simulink model "controlMCUCalibrateSurfaces"  (Simulink 6.6)
settings: Solver=FixedStepDiscrete  StartTime=0.0  StopTime=10.0  FixedStep=0.01  RelTol=1e-3
InitFcn:
  | mcuInit
undefined symbols (not defined in the file or in its folder): bdr, controlMCUInit, getPidIdx, gsRead, mdr, pilotCommands, prepareTelemetry, protParseDecode, protParseDecodeGS, readIpc, send2GS, u1, updateLoad, updatePWM, y1
libraries: dsPICdrivers x21, aerolibconvert2 x1, simulink x1
settings Model: Creator=ASL_Lab  LastModifiedBy=Administrator  ProdHWDeviceType=16-bit Generic
settings OptimizationCC: InlineParams=on  OptimizeModelRefInitCode=on  LifeSpan=1
settings HardwareCC: ProdBitPerInt=16  ProdEndianess=LittleEndian  ProdWordSize=16  ProdHWDeviceType=16-bit Generic  TargetHWDeviceType=32-bit Generic
settings RTWCC: SystemTargetFile=dspic.tlc  TemplateMakefile=dspic_pic30_gcc.tmf  PostCodeGenCommand=dsPIC_Compile()  Description=Embedded Target for Microchip dsPIC (real-time)  GenerateReport=on  ProcessScript=dspic_make_rtw_hook  IncludeHyperlinkInReport=on  LaunchReport=on
settings RTWCC: CustomSource=|
  | clib\circBuffer.c
  | clib\gpsSplit.c
  | clib\sbrk.c
  | clib\interProcCommSlave.c
  | clib\sendProtocol.c
  | clib\protDecoder.c
  | clib\groundStationDriver.c
  | clib\apUtils.c
  | clib\DEE.c
  | clib\DEES.s
  | clib\navSupport.c
settings CodeAppCC: IgnoreCustomStorageClasses=off
settings STFCustomTargetCC: TargetFcnLib=ansi_tfl_tmw.mat  GenFloatMathFcnCalls=ANSI_C  ModelReferenceCompliant=off  IncludeMdlTerminateFcn=off  CombineOutputUpdateFcns=on  SuppressErrorStatus=on  ERTCustomFileBanners=on  SupportContinuousTime=off  SupportNonInlinedSFcns=off  SystemTargetFile=dspic.tlc
settings ERTTargetCC: TargetFcnLib=ansi_tfl_tmw.mat  GenFloatMathFcnCalls=ANSI_C  ModelReferenceCompliant=off  IncludeMdlTerminateFcn=off  SuppressErrorStatus=on  ModelStepFunctionPrototypeControlCompliant=off  ExtModeMexFile=noextcomm  InlinedParameterPlacement=NonHierarchical  ERTSrcFileBannerTemplate=dsPIC_code_template.cgt  ERTHdrFileBannerTemplate=dsPIC_code_template.cgt  ERTDataSrcFileTemplate=dsPIC_code_template.cgt  ERTDataHdrFileTemplate=dsPIC_code_template.cgt  ERTCustomFileTemplate=dsPIC_main.tlc
settings CustomProperty: DataType=string  Value=C:\PROGRA~1\MATLAB\R2007a\rtw\bin\win32\gmake

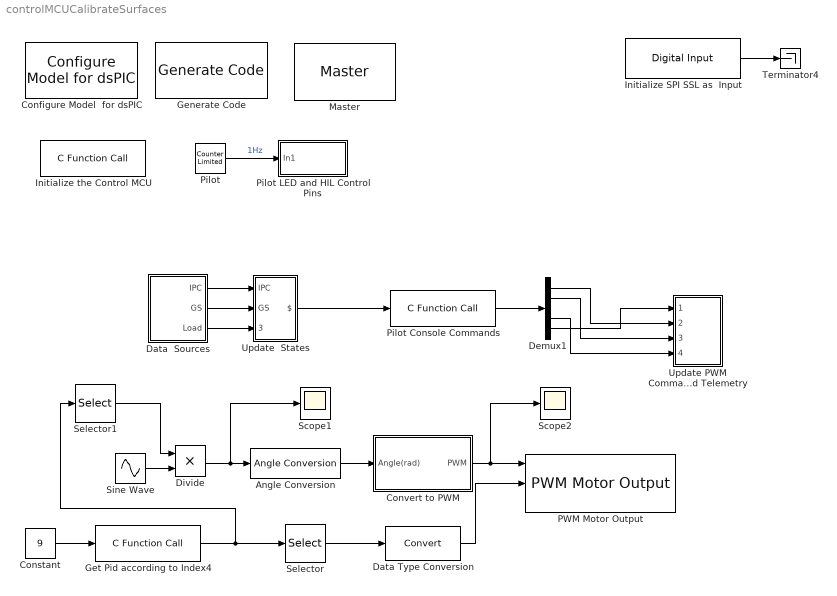
== system controlMCUCalibrateSurfaces ==
  Angle Conversion : aerolibconvert2/Angle Conversion  SystemSampleTime=-1  IU=deg  OU=rad
  Configure Model  for dsPIC : dsPICdrivers/Simulink Configuration/Configure Model  for dsPIC
  Constant : Constant  Value=9  OutDataTypeMode=uint8
  Convert to PWM : Subsystem  mask{slopem=mdr, interceptb=bdr}
      mask prompts: slopem "Slope"; interceptb "Intercept"
  Data  Sources : Subsystem
  Data Type Conversion : DataTypeConversion  OutDataTypeMode=uint16
  Demux1 : Demux  Outputs=5
  Divide : Product  OutScaling=2^-10
  Generate Code : dsPICdrivers/Simulink Configuration/Generate Code
  Get Pid according to Index4 : dsPICdrivers/OTHERS/C Function Call  Tag=dsPIC_dsPIC_CFunctionCall  fctName='getPidIdx'  INPUT_SIZE=1  INPUT1=uint8  INPUT2=--  INPUT3=--  OUTPUT_SIZE=3  OUTPUT1=real32  SampleTime=.01  InputType=[ 2 ]  OutputType=[ 7 ]  FctDeclaration=extern void getPidIdx(uint8_T u1,real32_T* y1);  FctCall=getPidIdx(%u1, *%y1);  OrderingInOutPopup=None
  Initialize SPI SSL as  Input : dsPICdrivers/Digital I//O/Digital Input  Tag=dsPIC_Digital_Input  PORT=B  Pin=[2]  SampleTime=inf  OrderingInOutPopup=None
  Initialize the Control MCU : dsPICdrivers/OTHERS/C Function Call  Tag=dsPIC_dsPIC_CFunctionCall  fctName='controlMCUInit'  INPUT_SIZE=1  INPUT1=--  INPUT2=--  INPUT3=--  OUTPUT_SIZE=1  OUTPUT1=--  SampleTime=inf  InputType=[ ]  OutputType=[ ]  FctDeclaration=extern void controlMCUInit();  FctCall=controlMCUInit();  OrderingInOutPopup=None
  Master : dsPICdrivers/Master  Tag=dsPIC_MASTER  Priority=1  TimeStepType=Timer1  picType=33fJ256MC710  fcy=40000000  Quartz_33f=12e6  PLLActive_33f=on  fcyDesired_33f=40e6  tmr1="[8  49999  0]"  tmr1Info="Time Step : 0.01  ;   Error : 0%  PR1=49999"  tmr2345="[0  0  0  0  0  0  0  0]"  tmr2345cfg=[-1 -1 -1 -1 -1 -1 -1 -1]  IOautoConf=on  typePort="[ 0   0   0   0   0   0   0   0   0   0   0   0   0   0   0   0   0   0   9   0   0   0  10  10   0   0   0   0   0   0   0   0   0   0   0   0   0   0   0   0   0   0   0   0   0   0   0   0   0   0   0   0   0   0   0   0   0   0   0   0   0   0   0   0  11   0   0   0  11   0  11   0   0  10   0   0   0   0   0   0   0   0   0   0   0   0   0   0   0   0   0   0   0   0   0   0   0   0   0   0   0   0   0   0   0   0   0   0   0   0   0   0 ]"  TRIS="[ 65535  65343  65535  65535  65023  65535  65535 ]"  ADPCFG=2097348  MasterBusyPort=None  MasterOverloadPort=None  FOSC=Quartz (XT - HS)  TempProtection_33f=TEMP_ON  FPBOR=<empty>  PWRT=64ms  MCLR=<empty>  PowerSave=off
  PWM Motor Output : dsPICdrivers/Peripheral I//O/PWM Motor Output  Tag=dsPIC_PWM_Motor  Priority=5  InputEnableChk=off  InputPeriodeChk=off  Channel=[1 3 4]  TPeriode=.02  PrescalerValue=16  PeriodeInteger=25000  MaxName='PWM'  Centered=on  HChannelON=off  Info="Nbr Bits : 15.6096  ||  PWM = 50000  ||  Prescaler = 16"  Delay=0  IntPriority=5  nbrPwmChannelPIC=4  Status=OK
  Pilot : simulink/Sources/Counter Limited  SystemSampleTime=-1  uplimit=1  tsamp=1.0
  Pilot Console Commands : dsPICdrivers/OTHERS/C Function Call  Tag=dsPIC_dsPIC_CFunctionCall  fctName='pilotCommands'  INPUT_SIZE=1  INPUT1=--  INPUT2=--  INPUT3=--  OUTPUT_SIZE=5  OUTPUT1=uint16  SampleTime=.01  InputType=[ ]  OutputType=[ 4 ]  FctDeclaration=extern void pilotCommands(uint16_T* y1);  FctCall=pilotCommands(*%y1);  OrderingInOutPopup=Input
  Pilot LED and HIL Control Pins : Subsystem
  Scope1 : Scope
  Scope2 : Scope
  Selector : Selector  IndexOptions=Index vector (dialog)  Indices=[1]  OutputSizes=1  InputPortWidth=3
  Selector1 : Selector  IndexOptions=Index vector (dialog)  Indices=[2]  OutputSizes=1  InputPortWidth=3
  Sine Wave : Sin  SineType=Sample based  Samples=250  SampleTime=0.01
  Terminator4 : Terminator
  Update  States : Subsystem
  Update PWM Commands and Send Telemetry : Subsystem
  wires:
  Initialize SPI SSL as  Input/1 -> Terminator4/1
  Pilot/1 -> Pilot LED and HIL Control Pins/1(In1)  "1Hz"
  Data  Sources/1(IPC) -> Update  States/1(IPC)
  Data  Sources/2(GS) -> Update  States/2(GS)
  Data  Sources/3(Load) -> Update  States/3(Load)
  Pilot Console Commands/1 -> Demux1/1
  Demux1/1 -> Update PWM Commands and Send Telemetry/2(dT (pwm))
  Demux1/2 -> Update PWM Commands and Send Telemetry/3(dA (pwm))
  Demux1/4 -> Update PWM Commands and Send Telemetry/4(dR (pwm))
  Demux1/5 -> Update PWM Commands and Send Telemetry/1(dE (pwm))
  Update  States/1($) -> Pilot Console Commands/1
  Convert to PWM/1(PWM) -> PWM Motor Output/1, Scope2/1
  Angle Conversion/1 -> Convert to PWM/1(" Angle(rad)")
  Constant/1 -> Get Pid according to Index4/1
  Get Pid according to Index4/1 -> Selector/1, Selector1/1
  Data Type Conversion/1 -> PWM Motor Output/2
  Selector/1 -> Data Type Conversion/1
  Sine Wave/1 -> Divide/2
  Divide/1 -> Angle Conversion/1, Scope1/1
  Selector1/1 -> Divide/1

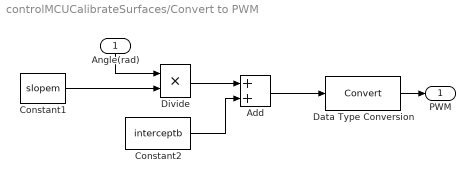
== system controlMCUCalibrateSurfaces/Convert to PWM ==
  " Angle(rad)" : Inport  Orientation=down
  Add : Sum  OutScaling=2^-10
  Constant1 : Constant  Value=slopem
  Constant2 : Constant  Value=interceptb
  Data Type Conversion : DataTypeConversion  OutDataTypeMode=uint16
  Divide : Product  OutScaling=2^-10
  PWM : Outport
  wires:
  Constant1/1 -> Divide/2
  Add/1 -> Data Type Conversion/1
  Divide/1 -> Add/1
  Constant2/1 -> Add/2
  " Angle(rad)"/1 -> Divide/1
  Data Type Conversion/1 -> PWM/1

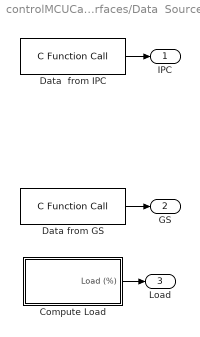
== system controlMCUCalibrateSurfaces/Data  Sources ==
  Compute Load : Subsystem
  Data from GS : dsPICdrivers/OTHERS/C Function Call  Tag=dsPIC_dsPIC_CFunctionCall  fctName='gsRead'  INPUT_SIZE=1  INPUT1=--  INPUT2=--  INPUT3=--  OUTPUT_SIZE=103  OUTPUT1=uint8  SampleTime=.01  InputType=[ ]  OutputType=[ 2 ]  FctDeclaration=extern void gsRead(uint8_T* y1);  FctCall=gsRead(*%y1);  OrderingInOutPopup=None
  Data  from IPC : dsPICdrivers/OTHERS/C Function Call  Tag=dsPIC_dsPIC_CFunctionCall  fctName='readIpc'  INPUT_SIZE=1  INPUT1=--  INPUT2=--  INPUT3=--  OUTPUT_SIZE=99  OUTPUT1=uint8  SampleTime=.01  InputType=[ ]  OutputType=[ 2 ]  FctDeclaration=extern void readIpc(uint8_T* y1);  FctCall=readIpc(*%y1);  OrderingInOutPopup=None
  IPC : Outport
  GS : Outport  Port=2
  Load : Outport  Port=3
  wires:
  Data  from IPC/1 -> IPC/1
  Data from GS/1 -> GS/1
  Compute Load/1(Load (%)) -> Load/1

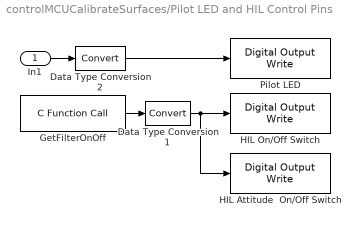
== system controlMCUCalibrateSurfaces/Pilot LED and HIL Control Pins ==
  In1 : Inport
  Data Type Conversion1 : DataTypeConversion  OutDataTypeMode=boolean
  Data Type Conversion2 : DataTypeConversion  OutDataTypeMode=boolean
  GetFilterOnOff : dsPICdrivers/OTHERS/C Function Call  Tag=dsPIC_dsPIC_CFunctionCall  fctName='getFilterOnOff'  INPUT_SIZE=1  INPUT1=--  INPUT2=--  INPUT3=--  OUTPUT_SIZE=1  OUTPUT1=uint8  SampleTime=.01  InputType=[ ]  OutputType=[ 2 ]  FctDeclaration=extern uint8_T getFilterOnOff();  FctCall=%y1 = getFilterOnOff();  OrderingInOutPopup=None
  HIL Attitude  On/Off Switch : dsPICdrivers/Digital I//O/Digital Output Write  Tag=dsPIC_Digital_Output  Priority=5  PORT=B  Pin=[6]  Simultaneous=off  OrderingInOutPopup=None
  HIL On/Off Switch : dsPICdrivers/Digital I//O/Digital Output Write  Tag=dsPIC_Digital_Output  Priority=5  PORT=E  Pin=[9]  Simultaneous=off  OrderingInOutPopup=None
  Pilot LED : dsPICdrivers/Digital I//O/Digital Output Write  Tag=dsPIC_Digital_Output  Priority=5  PORT=B  Pin=[ 7]  Simultaneous=off  OrderingInOutPopup=None
  wires:
  GetFilterOnOff/1 -> Data Type Conversion1/1
  Data Type Conversion1/1 -> HIL On/Off Switch/1, HIL Attitude  On/Off Switch/1
  Data Type Conversion2/1 -> Pilot LED/1
  In1/1 -> Data Type Conversion2/1

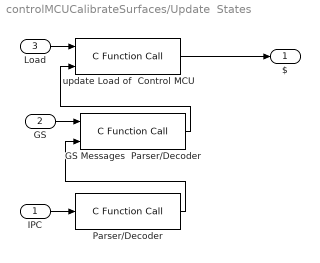
== system controlMCUCalibrateSurfaces/Update  States ==
  IPC : Inport
  GS : Inport  Port=2
  Load : Inport  Port=3
  GS Messages  Parser/Decoder : dsPICdrivers/OTHERS/C Function Call  Tag=dsPIC_dsPIC_CFunctionCall  fctName='protParseDecodeGS'  INPUT_SIZE=103  INPUT1=uint8  INPUT2=--  INPUT3=--  OUTPUT_SIZE=1  OUTPUT1=--  SampleTime=-1  InputType=[ 2 ]  OutputType=[ ]  FctDeclaration=extern void protParseDecodeGS(uint8_T* u1);  FctCall=protParseDecodeGS(*%u1);  OrderingInOutPopup=Input & Output
  Parser/Decoder : dsPICdrivers/OTHERS/C Function Call  Tag=dsPIC_dsPIC_CFunctionCall  fctName='protParseDecode'  INPUT_SIZE=99  INPUT1=uint8  INPUT2=--  INPUT3=--  OUTPUT_SIZE=1  OUTPUT1=--  SampleTime=-1  InputType=[ 2 ]  OutputType=[ ]  FctDeclaration=extern void protParseDecode(uint8_T* u1);  FctCall=protParseDecode(*%u1);  OrderingInOutPopup=Output
  update Load of  Control MCU : dsPICdrivers/OTHERS/C Function Call  Tag=dsPIC_dsPIC_CFunctionCall  fctName='updateLoad'  INPUT_SIZE=1  INPUT1=uint8  INPUT2=--  INPUT3=--  OUTPUT_SIZE=1  OUTPUT1=--  SampleTime=-1  InputType=[ 2 ]  OutputType=[ ]  FctDeclaration=extern void updateLoad(uint8_T u1);  FctCall=updateLoad(%u1);  OrderingInOutPopup=Input & Output
  $ : Outport
  wires:
  IPC/1 -> Parser/Decoder/1
  GS/1 -> GS Messages  Parser/Decoder/1
  Load/1 -> update Load of  Control MCU/1
  Parser/Decoder/1 -> GS Messages  Parser/Decoder/2
  GS Messages  Parser/Decoder/1 -> update Load of  Control MCU/2
  update Load of  Control MCU/1 -> $/1

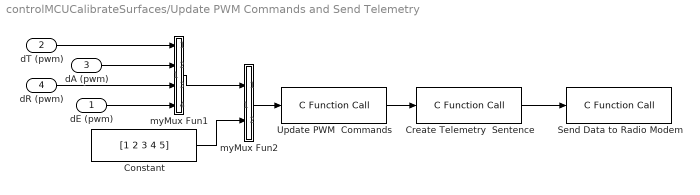
== system controlMCUCalibrateSurfaces/Update PWM Commands and Send Telemetry ==
  dE (pwm) : Inport
  dT (pwm) : Inport  Port=2
  dA (pwm) : Inport  Port=3
  dR (pwm) : Inport  Port=4
  Constant : Constant  Value=[1 2 3 4 5]  OutDataTypeMode=uint16  SampleTime=.01
  Create Telemetry  Sentence : dsPICdrivers/OTHERS/C Function Call  Tag=dsPIC_dsPIC_CFunctionCall  fctName='prepareTelemetry'  INPUT_SIZE=1  INPUT1=--  INPUT2=--  INPUT3=--  OUTPUT_SIZE=103  OUTPUT1=uint8  SampleTime=.01  InputType=[ ]  OutputType=[ 2 ]  FctDeclaration=extern void prepareTelemetry(uint8_T* y1);  FctCall=prepareTelemetry(*%y1);  OrderingInOutPopup=Input
  Send Data to Radio Modem : dsPICdrivers/OTHERS/C Function Call  Tag=dsPIC_dsPIC_CFunctionCall  fctName='send2GS'  INPUT_SIZE=103  INPUT1=uint8  INPUT2=--  INPUT3=--  OUTPUT_SIZE=1  OUTPUT1=--  SampleTime=-1  InputType=[ 2 ]  OutputType=[ ]  FctDeclaration=extern void send2GS(uint8_T* u1);  FctCall=send2GS(*%u1);  OrderingInOutPopup=None
  Update PWM  Commands : dsPICdrivers/OTHERS/C Function Call  Tag=dsPIC_dsPIC_CFunctionCall  fctName='updatePWM'  INPUT_SIZE=10  INPUT1=uint16  INPUT2=--  INPUT3=--  OUTPUT_SIZE=1  OUTPUT1=--  SampleTime=-1  InputType=[ 4 ]  OutputType=[ ]  FctDeclaration=extern void updatePWM(uint16_T* u1);  FctCall=updatePWM(*%u1);  OrderingInOutPopup=Output
  myMux Fun1 : Stateflow chart
  myMux Fun2 : Stateflow chart
  wires:
  Create Telemetry  Sentence/1 -> Send Data to Radio Modem/1
  Constant/1 -> myMux Fun2/2(u2)
  myMux Fun2/1(y) -> Update PWM  Commands/1
  myMux Fun1/1(y) -> myMux Fun2/1(u1)
  Update PWM  Commands/1 -> Create Telemetry  Sentence/1
  dT (pwm)/1 -> myMux Fun1/1(u1)
  dA (pwm)/1 -> myMux Fun1/2(u2)
  dR (pwm)/1 -> myMux Fun1/3(u3)
  dE (pwm)/1 -> myMux Fun1/4(u4)

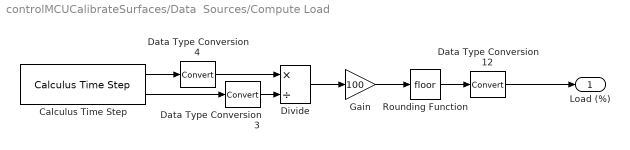
== system controlMCUCalibrateSurfaces/Data  Sources/Compute Load ==
  Calculus Time Step : dsPICdrivers/OTHERS/Calculus Time Step  Tag=dsPIC_CalculusTimeStep  SampleTime=0.01  PR1chk=on
  Data Type Conversion12 : DataTypeConversion  OutDataTypeMode=uint8
  Data Type Conversion3 : DataTypeConversion  OutDataTypeMode=single
  Data Type Conversion4 : DataTypeConversion  OutDataTypeMode=single
  Divide : Product  Inputs=*/  OutDataTypeMode=double  OutScaling=2^-10
  Gain : Gain  Gain=100
  Rounding Function : Rounding
  Load (%) : Outport
  wires:
  Calculus Time Step/1 -> Data Type Conversion4/1
  Calculus Time Step/2 -> Data Type Conversion3/1
  Divide/1 -> Gain/1
  Rounding Function/1 -> Data Type Conversion12/1
  Data Type Conversion3/1 -> Divide/2
  Data Type Conversion4/1 -> Divide/1
  Data Type Conversion12/1 -> Load (%)/1
  Gain/1 -> Rounding Function/1

== matlab function Update PWM Commands and Send Telemetry/myMux Fun1 ==
  data: u1 input inherited; y output inherited; u2 input inherited; u3 input inherited; u4 input inherited
function y = myMux(u1, u2, u3, u4 )
% This block supports an embeddable subset of the MATLAB language.
% See the help menu for details. 

y = [u1(1); u2(1); 0; u3(1); u4(1)];

== matlab function Update PWM Commands and Send Telemetry/myMux Fun2 ==
  data: u1 input inherited; y output inherited; u2 input inherited
function y = myMux(u1, u2)
% This block supports an embeddable subset of the MATLAB language.
% See the help menu for details. 

y = [u1(1:5); u2(1:5)];
